simulink model "S1"  (R2025a)
settings: Solver=VariableStepAuto  StartTime=0.0  StopTime=10.0  RelTol=1e-3
settings Model: Creator=a.diteodoro  LastModifiedBy=a.diteodoro

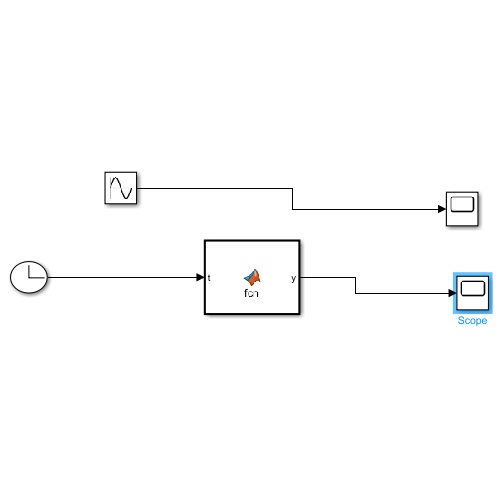
[thumbnail: Simulink's stored preview of the top-level diagram]
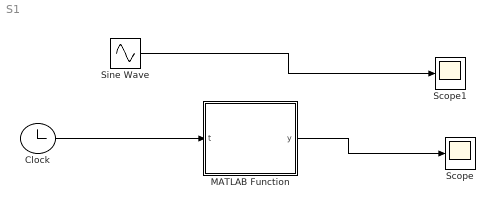
== system S1 ==
  Clock : Clock
  MATLAB Function : MATLAB Function  TreatAsAtomicUnit=on
  Scope : Scope
      settings: ActiveDisplayYMinimum=-12.431997361138825  ActiveDisplayYMaximum=111.88797625024945
  Scope1 : Scope
      settings: ActiveDisplayYMinimum=-1.2456318853205086  ActiveDisplayYMaximum=1.2490408795261734
  Sine Wave : Sin  SampleTime=0
  wires:
  Sine Wave/1 -> Scope1/1
  Clock/1 -> MATLAB Function/1(t)
  MATLAB Function/1(y) -> Scope/1

== matlab function S1/MATLAB Function ==
  data: t input; y output
function y = fcn(t)
y = sin(t) + t.^2;
